simulink model "Kinematics"  (R2022b)
settings: Solver=VariableStepAuto  StartTime=0.0  StopTime=10.0  RelTol=1e-3
settings Model: Creator=filippocamaleonte  LastModifiedBy=filippocamaleonte

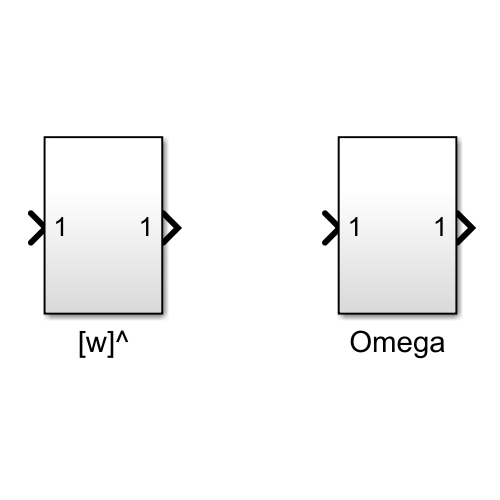
[thumbnail: Simulink's stored preview of the top-level diagram]
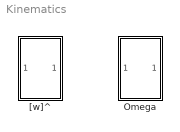
== system Kinematics ==
  Omega : Subsystem
  "[w]^" : Subsystem

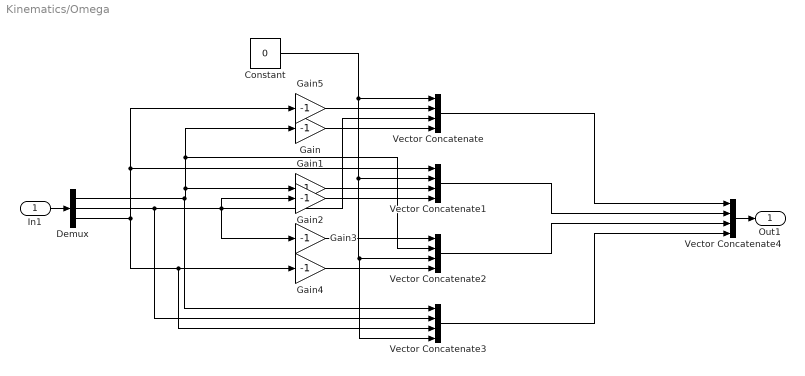
== system Kinematics/Omega ==
  In1 : Inport
  Constant : Constant  Value=0
  Demux : Demux  Outputs=3
  Gain{,1..5} (6 alike) : Gain  Gain=-1
  Vector Concatenate{,1..3} (4 alike) : Concatenate  NumInputs=4
  Vector Concatenate4 : Concatenate  NumInputs=4  Mode=Multidimensional array  ConcatenateDimension=2
  Out1 : Outport
  wires:
  Demux/2 -> Vector Concatenate3/2, Gain3/1, Gain2/1, Vector Concatenate/3
  Demux/3 -> Vector Concatenate3/3, Gain4/1, Vector Concatenate1/1, Gain5/1
  Vector Concatenate3/1 -> Vector Concatenate4/4
  Demux/1 -> Vector Concatenate3/1, Vector Concatenate2/2, Gain/1, Gain1/1
  Gain4/1 -> Vector Concatenate2/4
  Gain1/1 -> Vector Concatenate1/3
  Gain2/1 -> Vector Concatenate1/4
  Constant/1 -> Vector Concatenate3/4, Vector Concatenate2/3, Vector Concatenate1/2, Vector Concatenate/1
  Vector Concatenate/1 -> Vector Concatenate4/1
  Gain3/1 -> Vector Concatenate2/1
  Vector Concatenate2/1 -> Vector Concatenate4/3
  Vector Concatenate1/1 -> Vector Concatenate4/2
  Gain5/1 -> Vector Concatenate/2
  Gain/1 -> Vector Concatenate/4
  Vector Concatenate4/1 -> Out1/1
  In1/1 -> Demux/1

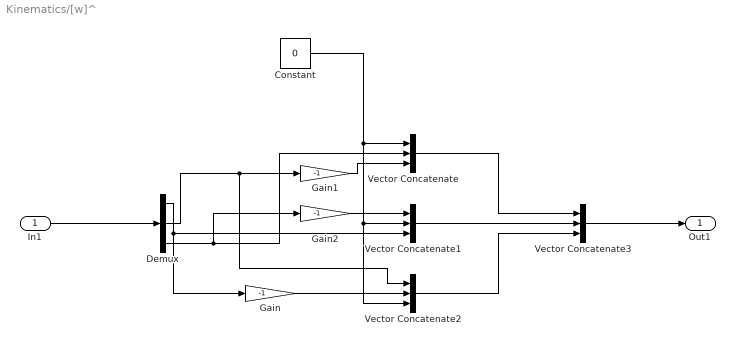
== system Kinematics/[w]^ ==
  In1 : Inport
  Constant : Constant  Value=0
  Demux : Demux  Outputs=3
  Gain : Gain  Gain=-1
  Gain1 : Gain  Gain=-1
  Gain2 : Gain  Gain=-1
  Vector Concatenate : Concatenate  NumInputs=3
  Vector Concatenate1 : Concatenate  NumInputs=3
  Vector Concatenate2 : Concatenate  NumInputs=3
  Vector Concatenate3 : Concatenate  NumInputs=3  Mode=Multidimensional array  ConcatenateDimension=2
  Out1 : Outport
  wires:
  Gain2/1 -> Vector Concatenate1/1
  Constant/1 -> Vector Concatenate2/3, Vector Concatenate1/2, Vector Concatenate/1
  Vector Concatenate2/1 -> Vector Concatenate3/3
  Vector Concatenate1/1 -> Vector Concatenate3/2
  Demux/2 -> Vector Concatenate2/1, Gain1/1
  Demux/1 -> Gain/1, Vector Concatenate1/3
  Vector Concatenate/1 -> Vector Concatenate3/1
  Demux/3 -> Gain2/1, Vector Concatenate/2
  Gain1/1 -> Vector Concatenate/3
  In1/1 -> Demux/1
  Gain/1 -> Vector Concatenate2/2
  Vector Concatenate3/1 -> Out1/1
